simulink model "New_FMS"  (R2018b)
settings: configuration reference "fms_config" (kept outside this file)
values from neighbouring files (symbols this model uses):
  FMS_PARAM = Simulink.Parameter(FMS_PARAM_VALUE)    [fms_model_init.m]
undefined symbols (not defined in the file or in its folder): actuator_cmd, ControlMode, DiscIntNeverNeededParam, FMS_Cmd, mode, MotionState, p_cmd, phi_cmd, PilotMode, psi_rate_cmd, q_cmd, r_cmd, reset, status, theta_cmd, throttle_cmd, u_cmd, v_cmd, VehicleStatus, w_cmd
libraries: FMT_Model_Lib x18, simulink x16
(part 1 of 3)
settings Model: Creator=jiachi  LastModifiedBy=jiachi
settings ConfigSetRef: SourceLocation=Base Workspace

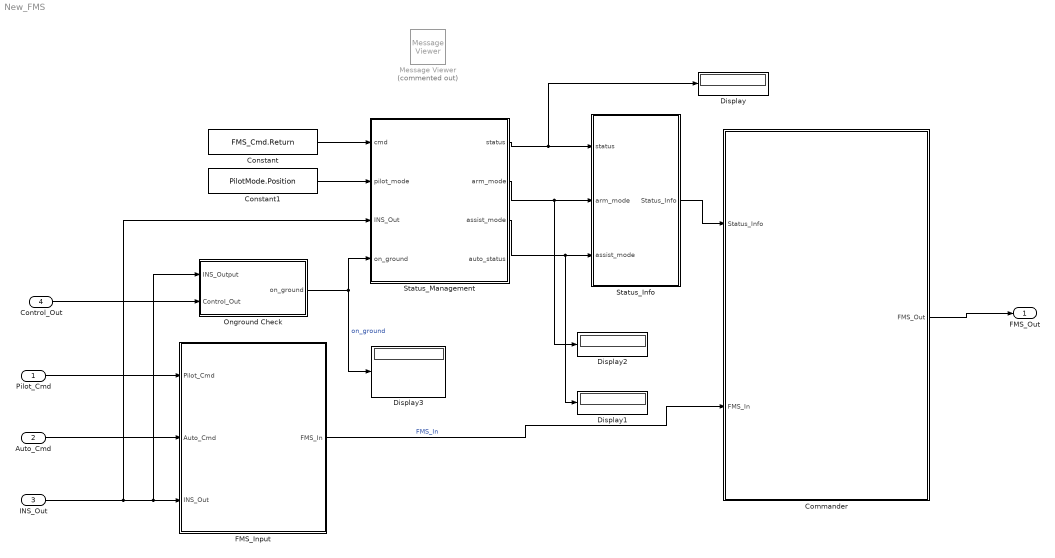
== system New_FMS ==
  Pilot_Cmd : Inport  OutDataTypeStr=Bus: Pilot_Cmd_Bus
  Auto_Cmd : Inport  Port=2  OutDataTypeStr=Bus: Auto_Cmd_Bus
  INS_Out : Inport  Port=3  OutDataTypeStr=Bus: INS_Out_Bus
  Control_Out : Inport  Port=4  OutDataTypeStr=Bus: Control_Out_Bus
  Commander : Subsystem
  Constant : Constant  Value=FMS_Cmd.Return  OutDataTypeStr=Enum: FMS_Cmd
  Constant1 : Constant  Value=PilotMode.Position  OutDataTypeStr=Enum: PilotMode
  Display{,1..3} (4 alike) : Display
  FMS_Input : Subsystem
  Message Viewer : MessageViewer  Commented=on  SavedRootId=#
  Onground Check : Subsystem
  Status_Info : Subsystem
  Status_Management : Stateflow chart  TreatAsAtomicUnit=on
  FMS_Out : Outport  OutDataTypeStr=Bus: FMS_Out_Bus
  wires:
  Status_Management/1(status) -> Status_Info/1(status), Display/1
  Constant/1 -> Status_Management/1(cmd)
  Commander/1(FMS_Out) -> FMS_Out/1
  Constant1/1 -> Status_Management/2(pilot_mode)
  Status_Management/2(arm_mode) -> Display2/1, Status_Info/2(arm_mode)
  Status_Management/3(assist_mode) -> Display1/1, Status_Info/3(assist_mode)
  Pilot_Cmd/1 -> FMS_Input/1(Pilot_Cmd)
  Auto_Cmd/1 -> FMS_Input/2(Auto_Cmd)
  INS_Out/1 -> Status_Management/3(INS_Out), Onground Check/1(INS_Output), FMS_Input/3(INS_Out)
  FMS_Input/1(FMS_In) -> Commander/2(FMS_In)  "FMS_In"
  Status_Info/1(Status_Info) -> Commander/1(Status_Info)
  Control_Out/1 -> Onground Check/2(Control_Out)
  Onground Check/1(on_ground) -> Display3/1, Status_Management/4(on_ground)  "on_ground"

== system New_FMS/Commander ==
  In Bus Element{3..4,6,9} (4 alike) : Inport  PortName=Status_Info
  In Bus Element2 : Inport  PortName=Status_Info  Element=vehicle_status
  In Bus Element{1,5,7..8} (4 alike) : Inport  Port=2  PortName=FMS_In
  Arm : Subsystem  TreatAsAtomicUnit=on
  Disarm : Subsystem  TreatAsAtomicUnit=on
  Land : Subsystem  TreatAsAtomicUnit=on
  Merge : Merge  Inputs=7
  Return : Subsystem  TreatAsAtomicUnit=on
  Standby : Subsystem  TreatAsAtomicUnit=on
  Status_Switch_Case : SwitchCase  CaseConditions={VehicleStatus.Disarm,VehicleStatus.Standby,VehicleStatus.Arm,VehicleStatus.Takeoff,VehicleStatus.Land,VehicleStatus.Return}
  Takeoff : Subsystem  TreatAsAtomicUnit=on
  Unknown : Subsystem  TreatAsAtomicUnit=on
  FMS_Out : Outport
  wires:
  Arm/1(FMS_Out) -> Merge/3
  Status_Switch_Case/6 -> Return/Action
  Takeoff/1(FMS_Out) -> Merge/4
  Status_Switch_Case/7 -> Unknown/Action
  Status_Switch_Case/2 -> Standby/Action
  Land/1(FMS_Out) -> Merge/5
  Unknown/1(FMS_Out) -> Merge/7
  Merge/1 -> FMS_Out/1
  Status_Switch_Case/1 -> Disarm/Action
  Status_Switch_Case/3 -> Arm/Action
  Status_Switch_Case/5 -> Land/Action
  Return/1(FMS_Out) -> Merge/6
  Status_Switch_Case/4 -> Takeoff/Action
  Disarm/1(FMS_Out) -> Merge/1
  Standby/1(FMS_Out) -> Merge/2
  In Bus Element3/1 -> Arm/1(Stauts_Info)
  In Bus Element1/1 -> Arm/2(FMS_In)
  In Bus Element2/1 -> Status_Switch_Case/1
  In Bus Element4/1 -> Takeoff/1(Status_Info)
  In Bus Element5/1 -> Takeoff/2(FMS_In)
  In Bus Element6/1 -> Land/1(Status_Info)
  In Bus Element7/1 -> Land/2(FMS_In)
  In Bus Element8/1 -> Return/2(FMS_In)
  In Bus Element9/1 -> Return/1(Status_Info)

== system New_FMS/FMS_Input ==
  Pilot_Cmd : Inport
  Auto_Cmd : Inport  Port=2
  INS_Out : Inport  Port=3
  Bus Creator : BusCreator  Inputs=4
  Bus Selector : BusSelector  OutputSignals=psi
  Pilot_Cmd_Process : Subsystem
  Psi To DCM : FMT_Model_Lib/Transformation/Psi To DCM
      settings: SourceProductName=FMT Toolbox
  Signal Copy : SignalConversion  OverrideOpt=off
  Signal Copy1 : SignalConversion  OverrideOpt=off
  FMS_In : Outport
  wires:
  Bus Creator/1 -> FMS_In/1
  Pilot_Cmd/1 -> Pilot_Cmd_Process/1(Pilot_Cmd)
  Auto_Cmd/1 -> Signal Copy/1
  INS_Out/1 -> Bus Selector/1, Signal Copy1/1  "INS_Out"
  Pilot_Cmd_Process/1(Pilot_Cmd_Proc) -> Bus Creator/1  "Pilot_Cmd_Proc"
  Bus Selector/1 -> Psi To DCM/1  "<psi>"
  Psi To DCM/1 -> Bus Creator/4  "M_CO"
  Signal Copy/1 -> Bus Creator/2  "Auto_Cmd"
  Signal Copy1/1 -> Bus Creator/3  "INS_Out"

== system New_FMS/Onground Check ==
  INS_Output : Inport
  Control_Out : Inport  Port=2
  Bus Selector1 : BusSelector  OutputSignals=actuator_cmd
  Bus Selector3 : BusSelector  OutputSignals=ax,ay,az
  Compare To Constant : simulink/Logic and Bit Operations/Compare To Constant  relop=<  const=1200  OutDataTypeStr=boolean
  Constant : Constant  Value=4  OutDataTypeStr=uint16
  Divide : Product  Inputs=*/
  First Order LPF : FMT_Model_Lib/Filter/First Order LPF  fc=1/(2*pi*0.5)
      settings: SourceProductName=FMT Toolbox
  First Order LPF1 : FMT_Model_Lib/Filter/First Order LPF  fc=1/(2*pi*0.1)
      settings: SourceProductName=FMT Toolbox
  Interval Test : simulink/Logic and Bit Operations/Interval Test  IntervalClosedRight=on  uplimit=[0.5, 0.5, -9.806+0.5]  IntervalClosedLeft=on  lowlimit=[-0.5, -0.5, -9.806-0.5]  OutDataTypeStr=boolean
  Logical Operator : Logic  Inputs=1  AllPortsSameDT=off  OutDataTypeStr=boolean
  Logical Operator1 : Logic  AllPortsSameDT=off  OutDataTypeStr=boolean
  Matrix Concatenate3 : Concatenate  NumInputs=3  ConcatenateDimension=2
  Selector : Selector  InputPortWidth=16  IndexOptions=Index vector (dialog)  Indices=[1:4]  OutputSizes=1
  Sum of Elements : Sum  Inputs=+
  sample_valid : Subsystem
  on_ground : Outport
  wires:
  Bus Selector3/2 -> Matrix Concatenate3/2  "<ay>"
  Compare To Constant/1 -> Logical Operator1/2
  Bus Selector3/3 -> Matrix Concatenate3/3  "<az>"
  Bus Selector1/1 -> Selector/1  "<actuator_cmd>"
  Bus Selector3/1 -> Matrix Concatenate3/1  "<ax>"
  Selector/1 -> Sum of Elements/1
  INS_Output/1 -> Bus Selector3/1
  Logical Operator1/1 -> sample_valid/1(valid)
  Control_Out/1 -> Bus Selector1/1
  Matrix Concatenate3/1 -> First Order LPF/1
  Interval Test/1 -> Logical Operator/1
  Sum of Elements/1 -> Divide/1
  Constant/1 -> Divide/2
  First Order LPF/1 -> Interval Test/1
  Divide/1 -> First Order LPF1/1
  First Order LPF1/1 -> Compare To Constant/1
  Logical Operator/1 -> Logical Operator1/1
  sample_valid/1(sample_valid) -> on_ground/1

== system New_FMS/Status_Info ==
  status : Inport
  arm_mode : Inport  Port=2
  assist_mode : Inport  Port=3
  Bus Creator : BusCreator  Inputs=3
  Signal Copy : SignalConversion  OverrideOpt=off
  Signal Copy1 : SignalConversion  OverrideOpt=off
  Signal Copy2 : SignalConversion  OverrideOpt=off
  Status_Info : Outport
  wires:
  status/1 -> Signal Copy/1
  arm_mode/1 -> Signal Copy1/1
  assist_mode/1 -> Signal Copy2/1
  Signal Copy/1 -> Bus Creator/1  "vehicle_status"
  Signal Copy1/1 -> Bus Creator/2  "arm_mode"
  Signal Copy2/1 -> Bus Creator/3  "assist_mode"
  Bus Creator/1 -> Status_Info/1

== system New_FMS/Commander/Arm ==
  In Bus Element2 : Inport  PortName=Stauts_Info
  In Bus Element : Inport  PortName=Stauts_Info  Element=arm_mode
  In Bus Element1 : Inport  Port=2  PortName=FMS_In
  Action Port : ActionPort  InitializeStates=reset  ActionType=case
  Assist : Subsystem  TreatAsAtomicUnit=on
  Auto : Subsystem  TreatAsAtomicUnit=on
  Manual : Subsystem  TreatAsAtomicUnit=on
  Merge : Merge  Inputs=4
  Switch Case : SwitchCase  CaseConditions={ArmMode.Manual, ArmMode.Assist, ArmMode.Auto}
  Unknown : Subsystem  TreatAsAtomicUnit=on
  FMS_Out : Outport
  wires:
  Merge/1 -> FMS_Out/1
  In Bus Element/1 -> Switch Case/1
  Switch Case/1 -> Manual/Action
  Switch Case/2 -> Assist/Action
  Switch Case/3 -> Auto/Action
  Switch Case/4 -> Unknown/Action
  Manual/1(FMS_Out) -> Merge/1
  Assist/1(FMS_Out) -> Merge/2
  Auto/1(FMS_Out) -> Merge/3
  Unknown/1(FMS_Out) -> Merge/4
  In Bus Element2/1 -> Assist/1(Stauts_Info)
  In Bus Element1/1 -> Assist/2(FMS_In)

== system New_FMS/Commander/Disarm ==
  Action Port : ActionPort  InitializeStates=reset  ActionType=case
  Bus Assignment : BusAssignment  AssignedSignals=reset,status,actuator_cmd
  Constant : Constant  Value=0  OutDataTypeStr=Bus: FMS_Out_Bus
  Constant1 : Constant  Value=VehicleStatus.Disarm  OutDataTypeStr=Inherit: Inherit via back propagation
  Constant2 : Constant  OutDataTypeStr=Inherit: Inherit via back propagation
  Constant3 : Constant  Value=[1000;1000;1000;1000]  VectorParams1D=off  OutDataTypeStr=Inherit: Inherit via back propagation
  Constant4 : Constant  Value=zeros(12,1)  OutDataTypeStr=Inherit: Inherit via back propagation
  Mux : Mux  Inputs=2
  FMS_Out : Outport
  wires:
  Constant/1 -> Bus Assignment/1
  Bus Assignment/1 -> FMS_Out/1
  Constant2/1 -> Bus Assignment/2
  Constant1/1 -> Bus Assignment/3
  Constant3/1 -> Mux/1
  Constant4/1 -> Mux/2
  Mux/1 -> Bus Assignment/4

== system New_FMS/Commander/Land ==
  In Bus Element4 : Inport  PortName=Status_Info  Element=vehicle_status
  In Bus Element1 : Inport  Port=2  PortName=FMS_In
  Action Port : ActionPort  InitializeStates=reset  ActionType=case
  Bus Assignment1 : BusAssignment  AssignedSignals=reset,status,mode,psi_rate_cmd,u_cmd,v_cmd,w_cmd
  Constant : Constant  Value=0  OutDataTypeStr=Inherit: Inherit via back propagation
  Constant1 : Constant  Value=0  OutDataTypeStr=Bus: FMS_Out_Bus
  Constant2 : Constant  Value=ControlMode.POSCTL  OutDataTypeStr=Inherit: Inherit via back propagation
  Constant3 : Constant  Value=0  OutDataTypeStr=Inherit: Inherit via back propagation
  Constant4 : Constant  Value=0.5  OutDataTypeStr=Inherit: Inherit via back propagation
  Constant5 : Constant  Value=[0; 0]  OutDataTypeStr=single
  Position Command : Subsystem
  FMS_Out : Outport
  wires:
  Constant1/1 -> Bus Assignment1/1
  Constant/1 -> Bus Assignment1/5
  Position Command/2(v_cmd_mPs) -> Bus Assignment1/7
  In Bus Element1/1 -> Position Command/1(FMS_In)
  In Bus Element4/1 -> Bus Assignment1/3
  Constant2/1 -> Bus Assignment1/4
  Constant3/1 -> Bus Assignment1/2
  Position Command/1(u_cmd_mPs) -> Bus Assignment1/6
  Bus Assignment1/1 -> FMS_Out/1
  Constant4/1 -> Bus Assignment1/8
  Constant5/1 -> Position Command/2(home_xy_R)

== system New_FMS/Commander/Return ==
  In Bus Element4 : Inport  PortName=Status_Info  Element=vehicle_status
  In Bus Element : Inport  Port=2  PortName=FMS_In
  In Bus Element3 : Inport  Port=2  PortName=FMS_In
  Action Port : ActionPort  InitializeStates=reset  ActionType=case
  Bus Assignment1 : BusAssignment  AssignedSignals=reset,status,mode,u_cmd,v_cmd,w_cmd,psi_rate_cmd
  Constant2 : Constant  Value=0  OutDataTypeStr=Bus: FMS_Out_Bus
  Constant3 : Constant  Value=ControlMode.POSCTL  OutDataTypeStr=Inherit: Inherit via back propagation
  Constant4 : Constant  Value=0  OutDataTypeStr=Inherit: Inherit via back propagation
  Heading Commander : Subsystem
  L1 : Constant  Value=10  OutDataTypeStr=single
  Subsystem : Subsystem
  Sum : Sum  Inputs=+-|
  Velocity Commander : Subsystem
  FMS_Out : Outport
  wires:
  Bus Assignment1/1 -> FMS_Out/1
  In Bus Element/1 -> Subsystem/1(In1)
  Constant4/1 -> Bus Assignment1/2
  Constant3/1 -> Bus Assignment1/4
  In Bus Element4/1 -> Bus Assignment1/3
  Constant2/1 -> Bus Assignment1/1
  Subsystem/1(P1) -> Sum/2, Velocity Commander/1(P1)
  Subsystem/2(P2) -> Velocity Commander/2(P2), Sum/1
  Subsystem/3(P3) -> Velocity Commander/3(P3)
  L1/1 -> Velocity Commander/4(L1)
  Velocity Commander/1(u_cmd) -> Bus Assignment1/5
  Velocity Commander/2(v_cmd) -> Bus Assignment1/6
  Velocity Commander/3(w_cmd) -> Bus Assignment1/7
  In Bus Element3/1 -> Heading Commander/2(FMS_In), Velocity Commander/5(FMS_In)
  Heading Commander/1(psi_rad_cmd) -> Bus Assignment1/8
  Sum/1 -> Heading Commander/1(P1P2)  "P1P2"

== system New_FMS/Commander/Standby ==
  Action Port : ActionPort  InitializeStates=reset  ActionType=case
  Bus Assignment : BusAssignment  AssignedSignals=reset,status,actuator_cmd
  Constant : Constant  Value=0  OutDataTypeStr=Bus: FMS_Out_Bus
  Constant1 : Constant  Value=VehicleStatus.Standby  OutDataTypeStr=Inherit: Inherit via back propagation
  Constant2 : Constant  OutDataTypeStr=Inherit: Inherit via back propagation
  Constant3 : Constant  Value=[1150;1150;1150;1150]  VectorParams1D=off  OutDataTypeStr=Inherit: Inherit via back propagation
  Constant4 : Constant  Value=zeros(12,1)  OutDataTypeStr=Inherit: Inherit via back propagation
  Mux : Mux  Inputs=2
  FMS_Out : Outport
  wires:
  Constant1/1 -> Bus Assignment/3
  Constant3/1 -> Mux/1
  Mux/1 -> Bus Assignment/4
  Constant4/1 -> Mux/2
  Bus Assignment/1 -> FMS_Out/1
  Constant2/1 -> Bus Assignment/2
  Constant/1 -> Bus Assignment/1

== system New_FMS/Commander/Takeoff ==
  In Bus Element4 : Inport  PortName=Status_Info  Element=vehicle_status
  In Bus Element1 : Inport  Port=2  PortName=FMS_In
  Action Port : ActionPort  InitializeStates=reset  ActionType=case
  Bus Assignment1 : BusAssignment  AssignedSignals=reset,status,mode,psi_rate_cmd,u_cmd,v_cmd,w_cmd
  Constant : Constant  Value=0  OutDataTypeStr=Inherit: Inherit via back propagation
  Constant1 : Constant  Value=0  OutDataTypeStr=Bus: FMS_Out_Bus
  Constant2 : Constant  Value=ControlMode.POSCTL  OutDataTypeStr=Inherit: Inherit via back propagation
  Constant3 : Constant  Value=0  OutDataTypeStr=Inherit: Inherit via back propagation
  Constant4 : Constant  Value=-0.5  OutDataTypeStr=Inherit: Inherit via back propagation
  Position Command : Subsystem
  FMS_Out : Outport
  wires:
  Bus Assignment1/1 -> FMS_Out/1
  Constant1/1 -> Bus Assignment1/1
  Constant/1 -> Bus Assignment1/5
  Constant3/1 -> Bus Assignment1/2
  In Bus Element4/1 -> Bus Assignment1/3
  Constant2/1 -> Bus Assignment1/4
  Position Command/1(u_cmd_mPs) -> Bus Assignment1/6
  Position Command/2(v_cmd_mPs) -> Bus Assignment1/7
  In Bus Element1/1 -> Position Command/1(FMS_In)
  Constant4/1 -> Bus Assignment1/8

== system New_FMS/Commander/Unknown ==
  Action Port : ActionPort  InitializeStates=reset  ActionType=default
  Bus Assignment : BusAssignment  AssignedSignals=reset,status,actuator_cmd
  Constant : Constant  Value=0  OutDataTypeStr=Bus: FMS_Out_Bus
  Constant1 : Constant  Value=VehicleStatus.Disarm  OutDataTypeStr=Inherit: Inherit via back propagation
  Constant2 : Constant  OutDataTypeStr=Inherit: Inherit via back propagation
  Constant3 : Constant  Value=[1000;1000;1000;1000]  VectorParams1D=off  OutDataTypeStr=Inherit: Inherit via back propagation
  Constant4 : Constant  Value=zeros(12,1)  OutDataTypeStr=Inherit: Inherit via back propagation
  Mux : Mux  Inputs=2
  FMS_Out : Outport
  wires:
  Constant/1 -> Bus Assignment/1
  Bus Assignment/1 -> FMS_Out/1
  Constant2/1 -> Bus Assignment/2
  Constant1/1 -> Bus Assignment/3
  Constant3/1 -> Mux/1
  Constant4/1 -> Mux/2
  Mux/1 -> Bus Assignment/4

== system New_FMS/FMS_Input/Pilot_Cmd_Process ==
  Pilot_Cmd : Inport
  Bus Creator : BusCreator  Inputs=8
  Bus Selector : BusSelector  OutputSignals=timestamp,mode,cmd_1,cmd_2,ls_lr,ls_ud,rs_lr,rs_ud
  Saturation{,1..3} (4 alike) : Saturate  UpperLimit=1  LowerLimit=-1
  Signal Copy{,1..3} (4 alike) : SignalConversion  OverrideOpt=off
  Pilot_Cmd_Proc : Outport
  wires:
  Pilot_Cmd/1 -> Bus Selector/1
  Bus Selector/1 -> Signal Copy/1  "<timestamp>"
  Signal Copy/1 -> Bus Creator/1  "timestamp_ms"
  Bus Selector/2 -> Signal Copy1/1  "<mode>"
  Signal Copy1/1 -> Bus Creator/2  "pilot_mode"
  Bus Selector/3 -> Signal Copy2/1  "<cmd_1>"
  Signal Copy2/1 -> Bus Creator/3  "event_cmd"
  Bus Selector/4 -> Signal Copy3/1  "<cmd_2>"
  Signal Copy3/1 -> Bus Creator/4  "stataus_cmd"
  Bus Selector/5 -> Saturation/1  "<ls_lr>"
  Bus Selector/6 -> Saturation1/1  "<ls_ud>"
  Bus Selector/7 -> Saturation2/1  "<rs_lr>"
  Bus Selector/8 -> Saturation3/1  "<rs_ud>"
  Saturation/1 -> Bus Creator/5  "stick_yaw"
  Saturation1/1 -> Bus Creator/6  "stick_throttle"
  Saturation2/1 -> Bus Creator/7  "stick_roll"
  Saturation3/1 -> Bus Creator/8  "stick_pitch"
  Bus Creator/1 -> Pilot_Cmd_Proc/1

== system New_FMS/Onground Check/sample_valid ==
  valid : Inport
  Add : Sum  AccumDataTypeStr=uint32
  Data Type Conversion : DataTypeConversion  OutDataTypeStr=uint32
  Delay : Delay  DelayLength=1  InitialCondition=0  ExternalReset=Falling
      settings: InputPortMap=u0,r5
  Saturation : Saturate  UpperLimit=10000  LowerLimit=0
  valid_samples : simulink/Logic and Bit Operations/Compare To Constant  relop=>  const=100  OutDataTypeStr=boolean
  sample_valid : Outport
  wires:
  Add/1 -> Saturation/1
  valid_samples/1 -> sample_valid/1
  Delay/1 -> Add/2
  valid/1 -> Data Type Conversion/1
  Data Type Conversion/1 -> Delay/2, Add/1
  Saturation/1 -> valid_samples/1, Delay/1

== system New_FMS/Commander/Arm/Assist ==
  In Bus Element{3..5,7,9} (5 alike) : Inport  PortName=Stauts_Info
  In Bus Element : Inport  PortName=Stauts_Info  Element=assist_mode
  In Bus Element{1..2,6,8} (4 alike) : Inport  Port=2  PortName=FMS_In
  Action Port : ActionPort  InitializeStates=reset  ActionType=case
  Acro : Subsystem  TreatAsAtomicUnit=on
  Altitude : Subsystem  TreatAsAtomicUnit=on
  Merge : Merge  Inputs=5
  Position : Subsystem  TreatAsAtomicUnit=on
  Stabilize : Subsystem  TreatAsAtomicUnit=on
  Switch Case : SwitchCase  CaseConditions={AssistMode.Acro, AssistMode.Stabilize, AssistMode.Altitude, AssistMode.Position}
  Unknown : Subsystem  TreatAsAtomicUnit=on
  FMS_Out : Outport
  wires:
  Merge/1 -> FMS_Out/1
  In Bus Element/1 -> Switch Case/1
  Switch Case/1 -> Acro/Action
  Switch Case/2 -> Stabilize/Action
  Switch Case/3 -> Altitude/Action
  Switch Case/4 -> Position/Action
  Switch Case/5 -> Unknown/Action
  Acro/1(FMS_Out) -> Merge/1
  Stabilize/1(FMS_Out) -> Merge/2
  Altitude/1(FMS_Out) -> Merge/3
  Position/1(FMS_Out) -> Merge/4
  Unknown/1(FMS_Out) -> Merge/5
  In Bus Element1/1 -> Stabilize/2(FMS_In)
  In Bus Element2/1 -> Altitude/2(FMS_In)
  In Bus Element3/1 -> Stabilize/1(Status_Info)
  In Bus Element4/1 -> Altitude/1(Status_Info)
  In Bus Element5/1 -> Position/1(Status_Info)
  In Bus Element6/1 -> Position/2(FMS_In)
  In Bus Element7/1 -> Acro/1(Status_Info)
  In Bus Element8/1 -> Acro/2(FMS_In)
  In Bus Element9/1 -> Unknown/1(Status_Info)

== system New_FMS/Commander/Arm/Auto ==
  Action Port : ActionPort  InitializeStates=reset  ActionType=case
  Bus Assignment : BusAssignment  AssignedSignals=reset,status,actuator_cmd
  Constant : Constant  Value=0  OutDataTypeStr=Bus: FMS_Out_Bus
  FMS_Out : Outport
  wires:
  Constant/1 -> Bus Assignment/1
  Bus Assignment/1 -> FMS_Out/1

== system New_FMS/Commander/Arm/Manual ==
  Action Port : ActionPort  InitializeStates=reset  ActionType=case
  Bus Assignment : BusAssignment  AssignedSignals=reset,status,actuator_cmd
  Constant : Constant  Value=0  OutDataTypeStr=Bus: FMS_Out_Bus
  FMS_Out : Outport
  wires:
  Constant/1 -> Bus Assignment/1
  Bus Assignment/1 -> FMS_Out/1

== system New_FMS/Commander/Arm/Unknown ==
  Action Port : ActionPort  InitializeStates=reset  ActionType=default
  Bus Assignment : BusAssignment  AssignedSignals=reset,status,actuator_cmd
  Constant : Constant  Value=0  OutDataTypeStr=Bus: FMS_Out_Bus
  FMS_Out : Outport
  wires:
  Bus Assignment/1 -> FMS_Out/1
  Constant/1 -> Bus Assignment/1

== system New_FMS/Commander/Land/Position Command ==
  FMS_In : Inport
  home_xy_R : Inport  Port=2
  Demux : Demux  Outputs=2
  Position Control : Subsystem
  Saturation1 : Saturate  UpperLimit=FMS_PARAM.VEL_XY_LIM  LowerLimit=-FMS_PARAM.VEL_XY_LIM
  u_cmd_mPs : Outport
  v_cmd_mPs : Outport  Port=2
  wires:
  FMS_In/1 -> Position Control/1(FMS_In)
  Saturation1/1 -> Demux/1
  Demux/1 -> u_cmd_mPs/1
  Demux/2 -> v_cmd_mPs/1
  Position Control/1(uv_cmd_mPs) -> Saturation1/1
  home_xy_R/1 -> Position Control/2(home_xy_R)

== system New_FMS/Commander/Return/Heading Commander ==
  P1P2 : Inport
  FMS_In : Inport  Port=2
  Heading Control : Subsystem
  Included Angle : Subsystem
  North : Constant  Value=[1 0]  OutDataTypeStr=single
  psi_rad_cmd : Outport
  wires:
  Heading Control/1(psi_rate_cmd_radPs) -> psi_rad_cmd/1
  Included Angle/1(angle_rad) -> Heading Control/2(psi_cmd_rad)
  North/1 -> Included Angle/1(vec1)
  FMS_In/1 -> Heading Control/1(FMS_In)
  P1P2/1 -> Included Angle/2(vec2)

== system New_FMS/Commander/Return/Subsystem ==
  In1 : Inport
  Bus Selector : BusSelector  OutputSignals=INS_Out.x_R,INS_Out.y_R
  Constant1 : Constant  Value=[0 0]  OutDataTypeStr=single
  Delay : Delay  DelayLength=1  InitialConditionSource=Input port
      settings: InputPortMap=u0,p4
  Mux : Mux  Inputs=2
  P1 : Outport
  P2 : Outport  Port=2
  P3 : Outport  Port=3
  wires:
  Constant1/1 -> P2/1  "P2"
  In1/1 -> Bus Selector/1
  Delay/1 -> P1/1, Delay/1  "P1"
  Mux/1 -> P3/1, Delay/2  "P3"
  Bus Selector/1 -> Mux/1  "<x_R>"
  Bus Selector/2 -> Mux/2  "<y_R>"

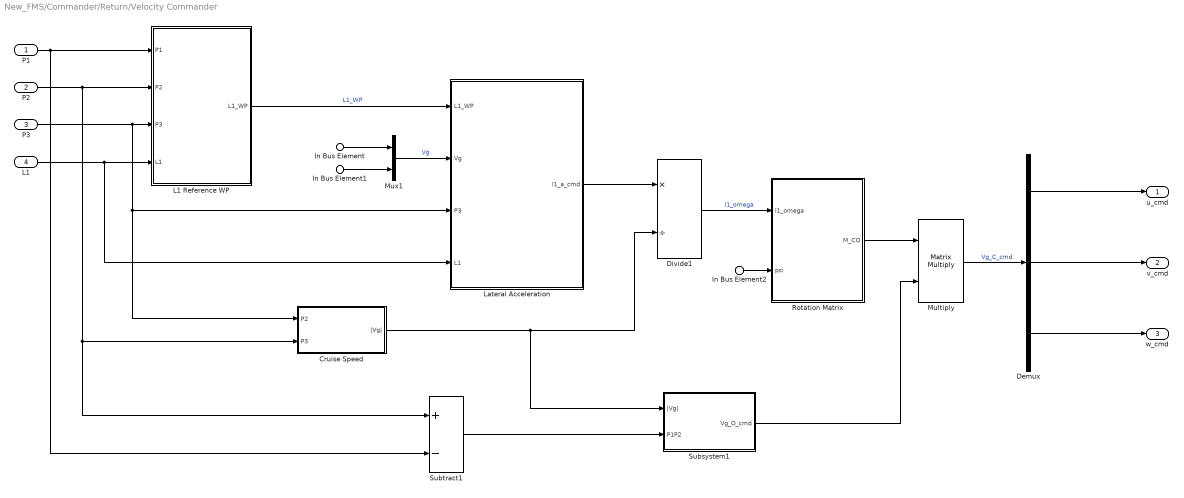
== system New_FMS/Commander/Return/Velocity Commander ==
  P1 : Inport
  P2 : Inport  Port=2
  P3 : Inport  Port=3
  L1 : Inport  Port=4
  In Bus Element : Inport  Port=5  PortName=FMS_In  Element=INS_Out.vn
  In Bus Element1 : Inport  Port=5  PortName=FMS_In  Element=INS_Out.ve
  In Bus Element2 : Inport  Port=5  PortName=FMS_In  Element=INS_Out.psi
  "Cruise Speed " : Subsystem
  Demux : Demux  Outputs=3
  Divide1 : Product  Inputs=*/
  L1 Reference WP : Subsystem
  Lateral Acceleration : Subsystem
  Multiply : Product  Multiplication=Matrix(*)
  Mux1 : Mux  Inputs=2
  Rotation Matrix : Subsystem
  Subsystem1 : Subsystem
  Subtract1 : Sum  Inputs=+-
  u_cmd : Outport
  v_cmd : Outport  Port=2
  w_cmd : Outport  Port=3
  wires:
  "Cruise Speed "/1(|Vg|) -> Divide1/2, Subsystem1/1(|Vg|)
  In Bus Element2/1 -> Rotation Matrix/2(psi)
  L1/1 -> L1 Reference WP/4(L1), Lateral Acceleration/4(L1)
  P1/1 -> Subtract1/2, L1 Reference WP/1(P1)
  L1 Reference WP/1(L1_WP) -> Lateral Acceleration/1(L1_WP)  "L1_WP"
  In Bus Element/1 -> Mux1/1
  Rotation Matrix/1(M_CO) -> Multiply/1
  Multiply/1 -> Demux/1  "Vg_C_cmd"
  Demux/1 -> u_cmd/1
  Demux/3 -> w_cmd/1
  Demux/2 -> v_cmd/1
  P2/1 -> L1 Reference WP/2(P2), Subtract1/1, "Cruise Speed "/2(P3)
  Mux1/1 -> Lateral Acceleration/2(Vg)  "Vg"
  Divide1/1 -> Rotation Matrix/1(l1_omega)  "l1_omega"
  In Bus Element1/1 -> Mux1/2
  P3/1 -> Lateral Acceleration/3(P3), "Cruise Speed "/1(P2), L1 Reference WP/3(P3)
  Subsystem1/1(Vg_O_cmd) -> Multiply/2
  Subtract1/1 -> Subsystem1/2(P1P2)
  Lateral Acceleration/1(l1_a_cmd) -> Divide1/1

== system New_FMS/Commander/Takeoff/Position Command ==
  FMS_In : Inport
  Constant : Constant  Value=MotionState.Hold  OutDataTypeStr=Enum: MotionState
  Controller : Subsystem
  Demux : Demux  Outputs=2
  u_cmd_mPs : Outport
  v_cmd_mPs : Outport  Port=2
  wires:
  FMS_In/1 -> Controller/2(FMS_In)
  Controller/1(uv_cmd_mPs) -> Demux/1
  Demux/1 -> u_cmd_mPs/1
  Demux/2 -> v_cmd_mPs/1
  Constant/1 -> Controller/1(motion_state)

== system New_FMS/Commander/Arm/Assist/Acro ==
  In Bus Element4 : Inport  PortName=Status_Info  Element=vehicle_status
  In Bus Element2 : Inport  Port=2  PortName=FMS_In  Element=Pilot_Cmd_Proc.stick_throttle
  In Bus Element1 : Inport  Port=2  PortName=FMS_In  Element=Pilot_Cmd_Proc.stick_pitch
  In Bus Element3 : Inport  Port=2  PortName=FMS_In  Element=Pilot_Cmd_Proc.stick_roll
  In Bus Element5 : Inport  Port=2  PortName=FMS_In  Element=Pilot_Cmd_Proc.stick_yaw
  Action Port : ActionPort  InitializeStates=reset  ActionType=case
  Angular Rate Command : Subsystem
  Bus Assignment : BusAssignment  AssignedSignals=reset,status,mode,p_cmd,q_cmd,r_cmd,throttle_cmd
  Constant : Constant  Value=0  OutDataTypeStr=Bus: FMS_Out_Bus
  Constant1 : Constant  Value=0  OutDataTypeStr=Inherit: Inherit via back propagation
  Constant2 : Constant  Value=ControlMode.Acro  OutDataTypeStr=Inherit: Inherit via back propagation
  Throttle Command : Subsystem
  FMS_Out : Outport
  wires:
  Constant1/1 -> Bus Assignment/2
  Constant2/1 -> Bus Assignment/4
  Angular Rate Command/3(r_cmd_radPs) -> Bus Assignment/7
  Bus Assignment/1 -> FMS_Out/1
  Constant/1 -> Bus Assignment/1
  Angular Rate Command/1(p_cmd_radPs) -> Bus Assignment/5
  Angular Rate Command/2(q_cmd_radPs) -> Bus Assignment/6
  Throttle Command/1(throttle_cmd) -> Bus Assignment/8
  In Bus Element4/1 -> Bus Assignment/3
  In Bus Element2/1 -> Throttle Command/1(stick_throttle)
  In Bus Element5/1 -> Angular Rate Command/3(stick_yaw)
  In Bus Element1/1 -> Angular Rate Command/2(stick_pitch)
  In Bus Element3/1 -> Angular Rate Command/1(stick_roll)

== system New_FMS/Commander/Arm/Assist/Altitude ==
  In Bus Element4 : Inport  PortName=Status_Info  Element=vehicle_status
  In Bus Element3 : Inport  Port=2  PortName=FMS_In
  In Bus Element5 : Inport  Port=2  PortName=FMS_In
  In Bus Element1 : Inport  Port=2  PortName=FMS_In  Element=Pilot_Cmd_Proc.stick_roll
  In Bus Element2 : Inport  Port=2  PortName=FMS_In  Element=Pilot_Cmd_Proc.stick_pitch
  Action Port : ActionPort  InitializeStates=reset  ActionType=case
  Altitude Command : Subsystem
  Attitude Command : Subsystem
  Bus Assignment : BusAssignment  AssignedSignals=reset,status,mode,phi_cmd,theta_cmd,psi_rate_cmd,w_cmd
  Constant : Constant  Value=0  OutDataTypeStr=Bus: FMS_Out_Bus
  Constant2 : Constant  Value=ControlMode.ALTCTL  OutDataTypeStr=Inherit: Inherit via back propagation
  Constant3 : Constant  Value=0  OutDataTypeStr=Inherit: Inherit via back propagation
  Heading Command : Subsystem
  FMS_Out : Outport
  wires:
  Constant/1 -> Bus Assignment/1
  Bus Assignment/1 -> FMS_Out/1
  In Bus Element4/1 -> Bus Assignment/3
  Constant2/1 -> Bus Assignment/4
  In Bus Element1/1 -> Attitude Command/1(stick_roll)
  In Bus Element2/1 -> Attitude Command/2(stick_pitch)
  In Bus Element3/1 -> Heading Command/1(FMS_In)
  Altitude Command/1(w_cmd_mPs) -> Bus Assignment/8
  Constant3/1 -> Bus Assignment/2
  Attitude Command/1(phi_cmd_radPs) -> Bus Assignment/5
  Attitude Command/2(theta_cmd_radPs) -> Bus Assignment/6
  Heading Command/1(psi_rate_cmd_radPs) -> Bus Assignment/7
  In Bus Element5/1 -> Altitude Command/1(FMS_In)

== system New_FMS/Commander/Arm/Assist/Position ==
  In Bus Element4 : Inport  PortName=Status_Info  Element=vehicle_status
  In Bus Element3 : Inport  Port=2  PortName=FMS_In
  In Bus Element5 : Inport  Port=2  PortName=FMS_In
  In Bus Element1 : Inport  Port=2  PortName=FMS_In
  Action Port : ActionPort  InitializeStates=reset  ActionType=case
  Altitude Command : Subsystem
  Bus Assignment : BusAssignment  AssignedSignals=reset,status,mode,psi_rate_cmd,u_cmd,v_cmd,w_cmd
  Constant : Constant  Value=0  OutDataTypeStr=Bus: FMS_Out_Bus
  Constant2 : Constant  Value=ControlMode.POSCTL  OutDataTypeStr=Inherit: Inherit via back propagation
  Constant3 : Constant  Value=0  OutDataTypeStr=Inherit: Inherit via back propagation
  Heading Command : Subsystem
  Position Command : Subsystem
  FMS_Out : Outport
  wires:
  Bus Assignment/1 -> FMS_Out/1
  Constant/1 -> Bus Assignment/1
  Constant3/1 -> Bus Assignment/2
  In Bus Element4/1 -> Bus Assignment/3
  Constant2/1 -> Bus Assignment/4
  Heading Command/1(psi_rate_cmd_radPs) -> Bus Assignment/5
  In Bus Element3/1 -> Heading Command/1(FMS_In)
  Altitude Command/1(w_cmd_mPs) -> Bus Assignment/8
  In Bus Element5/1 -> Altitude Command/1(FMS_In)
  In Bus Element1/1 -> Position Command/1(FMS_In)
  Position Command/1(u_cmd_mPs) -> Bus Assignment/6
  Position Command/2(v_cmd_mPs) -> Bus Assignment/7

== system New_FMS/Commander/Arm/Assist/Stabilize ==
  In Bus Element4 : Inport  PortName=Status_Info  Element=vehicle_status
  In Bus Element3 : Inport  Port=2  PortName=FMS_In
  In Bus Element1 : Inport  Port=2  PortName=FMS_In  Element=Pilot_Cmd_Proc.stick_roll
  In Bus Element2 : Inport  Port=2  PortName=FMS_In  Element=Pilot_Cmd_Proc.stick_pitch
  In Bus Element : Inport  Port=2  PortName=FMS_In  Element=Pilot_Cmd_Proc.stick_throttle
  Action Port : ActionPort  InitializeStates=reset  ActionType=case
  Attitude Command : Subsystem
  Bus Assignment : BusAssignment  AssignedSignals=reset,status,mode,phi_cmd,theta_cmd,psi_rate_cmd,throttle_cmd
  Constant : Constant  Value=0  OutDataTypeStr=Bus: FMS_Out_Bus
  Constant1 : Constant  Value=0  OutDataTypeStr=Inherit: Inherit via back propagation
  Constant2 : Constant  Value=ControlMode.Stabilize  OutDataTypeStr=Inherit: Inherit via back propagation
  Heading Command : Subsystem
  Throttle Command : Subsystem
  FMS_Out : Outport
  wires:
  Bus Assignment/1 -> FMS_Out/1
  Constant/1 -> Bus Assignment/1
  Constant1/1 -> Bus Assignment/2
  Constant2/1 -> Bus Assignment/4
  Heading Command/1(psi_rate_cmd_radPs) -> Bus Assignment/7
  Attitude Command/1(phi_cmd_radPs) -> Bus Assignment/5
  Attitude Command/2(theta_cmd_radPs) -> Bus Assignment/6
  In Bus Element1/1 -> Attitude Command/1(stick_roll)
  In Bus Element2/1 -> Attitude Command/2(stick_pitch)
  In Bus Element/1 -> Throttle Command/1(stick_throttle)
  Throttle Command/1(throttle_cmd) -> Bus Assignment/8
  In Bus Element3/1 -> Heading Command/1(FMS_In)
  In Bus Element4/1 -> Bus Assignment/3

== system New_FMS/Commander/Arm/Assist/Unknown ==
  In Bus Element4 : Inport  PortName=Status_Info  Element=vehicle_status
  Action Port : ActionPort  InitializeStates=reset  ActionType=default
  Bus Assignment : BusAssignment  AssignedSignals=reset,status,mode,actuator_cmd
  Constant : Constant  Value=0  OutDataTypeStr=Bus: FMS_Out_Bus
  Constant1 : Constant  OutDataTypeStr=Inherit: Inherit via back propagation
  Constant2 : Constant  Value=ControlMode.Unknown  OutDataTypeStr=Inherit: Inherit via back propagation
  Constant3 : Constant  Value=zeros(16,1)  OutDataTypeStr=Inherit: Inherit via back propagation
  FMS_Out : Outport
  wires:
  Constant/1 -> Bus Assignment/1
  Bus Assignment/1 -> FMS_Out/1
  Constant1/1 -> Bus Assignment/2
  Constant2/1 -> Bus Assignment/4
  In Bus Element4/1 -> Bus Assignment/3
  Constant3/1 -> Bus Assignment/5

== system New_FMS/Commander/Land/Position Command/Position Control ==
  FMS_In : Inport
  home_xy_R : Inport  Port=2
  Bus Selector : BusSelector  OutputSignals=INS_Out.psi
  Bus_Selection : Subsystem
  Constant : Constant  Value=0  OutDataTypeStr=Inherit: Inherit via back propagation
  Gain2 : Gain  Gain=FMS_PARAM.XY_P  OutDataTypeStr=single
  Multiply : Product  Multiplication=Matrix(*)
  Mux : Mux  Inputs=2
  Psi To DCM : FMT_Model_Lib/Transformation/Psi To DCM
      settings: SourceProductName=FMT Toolbox
  Selector : Selector  InputPortWidth=3  IndexOptions=Index vector (dialog)  Indices=[1 2]  OutputSizes=1
  Sum : Sum  Inputs=-+|
  uv_cmd_mPs : Outport
  wires:
  Gain2/1 -> uv_cmd_mPs/1
  Bus_Selection/1(xy_R_O_m) -> Sum/1  "xy_est_R"
  Sum/1 -> Mux/1  "xy_err_R"
  home_xy_R/1 -> Sum/2
  FMS_In/1 -> Bus Selector/1, Bus_Selection/1(FMS_In)
  Constant/1 -> Mux/2
  Psi To DCM/1 -> Multiply/1  "M_CO"
  Multiply/1 -> Selector/1
  Mux/1 -> Multiply/2
  Selector/1 -> Gain2/1
  Bus Selector/1 -> Psi To DCM/1  "<psi>"

== system New_FMS/Commander/Return/Heading Commander/Heading Control ==
  FMS_In : Inport
  psi_cmd_rad : Inport  Port=2
  Bus Selector : BusSelector  OutputSignals=INS_Out.psi
  Heading Control : Subsystem  TreatAsAtomicUnit=on
  TD : Subsystem
  psi_rate_cmd_radPs : Outport
  wires:
  TD/1(v1) -> Heading Control/2(psi_cmd_rad)
  FMS_In/1 -> Bus Selector/1, Heading Control/1(FMS_In)
  Bus Selector/1 -> TD/2(v0)  "<psi>"
  Heading Control/1(psi_rate_cmd_radPs) -> psi_rate_cmd_radPs/1
  psi_cmd_rad/1 -> TD/1(v)

== system New_FMS/Commander/Return/Heading Commander/Included Angle ==
  vec1 : Inport
  vec2 : Inport  Port=2
  2D Cross Product : FMT_Model_Lib/Math/2D Cross Product
      settings: SourceProductName=FMT Toolbox
  Acos : Trigonometry  Operator=acos
  Constant4 : Constant  OutDataTypeStr=single
  Demux : Demux  Outputs=2
  Demux1 : Demux  Outputs=2
  Dot Product : DotProduct  InputSameDT=on  OutDataTypeStr=Inherit: Inherit via internal rule
  Multiply : Product
  Mux : Mux  Inputs=2
  Mux1 : Mux  Inputs=2
  Sign1 : Signum
  Switch2 : Switch  Criteria=u2 ~= 0
  Vector Normalize : FMT_Model_Lib/Math/Vector Normalize
      settings: SourceProductName=FMT Toolbox
  Vector Normalize1 : FMT_Model_Lib/Math/Vector Normalize
      settings: SourceProductName=FMT Toolbox
  angle_rad : Outport
  wires:
  Dot Product/1 -> Acos/1
  Demux1/1 -> Mux1/2
  Mux1/1 -> Vector Normalize/1
  Demux1/2 -> Mux1/1
  Sign1/1 -> Switch2/1, Switch2/2
  Vector Normalize1/1 -> Dot Product/2, 2D Cross Product/1
  Demux/2 -> Mux/1
  Vector Normalize/1 -> Dot Product/1, 2D Cross Product/2
  2D Cross Product/1 -> Sign1/1
  Multiply/1 -> angle_rad/1
  vec1/1 -> Demux1/1
  Demux/1 -> Mux/2
  Constant4/1 -> Switch2/3
  vec2/1 -> Demux/1
  Mux/1 -> Vector Normalize1/1
  Acos/1 -> Multiply/1
  Switch2/1 -> Multiply/2

== system New_FMS/Commander/Return/Velocity Commander/Cruise Speed  ==
  P2 : Inport
  P3 : Inport  Port=2
  Gain : Gain  Gain=0.5  OutDataTypeStr=Inherit: Same as input
  Sum : Sum  Inputs=|+-
  Switch : Switch  Criteria=u2 > Threshold  Threshold=10
  Vector Modulus : FMT_Model_Lib/Math/Vector Modulus
      settings: SourceProductName=FMT Toolbox
  vel : Constant  Value=5  OutDataTypeStr=single
  |Vg| : Outport
  wires:
  P2/1 -> Sum/1
  P3/1 -> Sum/2
  Sum/1 -> Vector Modulus/1
  Vector Modulus/1 -> Gain/1, Switch/2
  vel/1 -> Switch/1  "|Vg|"
  Switch/1 -> |Vg|/1
  Gain/1 -> Switch/3

== system New_FMS/Commander/Return/Velocity Commander/L1 Reference WP ==
  P1 : Inport
  P2 : Inport  Port=2
  P3 : Inport  Port=3
  L1 : Inport  Port=4
  Compare To Constant : simulink/Logic and Bit Operations/Compare To Constant  relop=>=  const=0  OutDataTypeStr=boolean
  Compare To Constant1 : simulink/Logic and Bit Operations/Compare To Constant  relop=>  const=0  OutDataTypeStr=boolean
  NearbyRefWP : MATLAB Function  TreatAsAtomicUnit=on
  OutRegionRegWP : MATLAB Function  TreatAsAtomicUnit=on
  SearchL1RefWP : MATLAB Function  TreatAsAtomicUnit=on
  Switch : Switch  Criteria=u2 > Threshold
  Switch1 : Switch  Criteria=u2 > Threshold
  L1_WP : Outport
  wires:
  NearbyRefWP/1(P) -> Switch1/1  "NearbyWP"
  SearchL1RefWP/1(P) -> Switch/1  "L1_Ref_P"
  Switch1/1 -> L1_WP/1
  OutRegionRegWP/1(P) -> Switch/3  "out_WP"
  L1/1 -> NearbyRefWP/3(L1), SearchL1RefWP/4(L1)
  Switch/1 -> Switch1/3
  P3/1 -> OutRegionRegWP/3(P3), SearchL1RefWP/3(P3), NearbyRefWP/2(P3)
  P2/1 -> OutRegionRegWP/2(P2), NearbyRefWP/1(P2), SearchL1RefWP/2(P2)
  P1/1 -> OutRegionRegWP/1(P1), SearchL1RefWP/1(P1)
  Compare To Constant1/1 -> Switch1/2
  SearchL1RefWP/2(u) -> Compare To Constant/1  "l1_u"
  NearbyRefWP/2(d) -> Compare To Constant1/1  "distance"
  Compare To Constant/1 -> Switch/2

== system New_FMS/Commander/Return/Velocity Commander/Lateral Acceleration ==
  L1_WP : Inport
  Vg : Inport  Port=2
  P3 : Inport  Port=3
  L1 : Inport  Port=4
  Divide : Product  Inputs=*/
  Gain : Gain  Gain=2
  Included Angle : Subsystem
  Multiply1 : Product
  Saturation : Saturate  UpperLimit=pi/2  LowerLimit=-pi/2
  Sin : Trigonometry
  Square : Math  Operator=square  SaturateOnIntegerOverflow=on
  Subtract : Sum  Inputs=+-
  Vector Modulus : FMT_Model_Lib/Math/Vector Modulus
      settings: SourceProductName=FMT Toolbox
  Vector Normalize : FMT_Model_Lib/Math/Vector Normalize
      settings: SourceProductName=FMT Toolbox
  Vector Normalize1 : FMT_Model_Lib/Math/Vector Normalize
      settings: SourceProductName=FMT Toolbox
  l1_a_cmd : Outport
  wires:
  P3/1 -> Subtract/2
  Sin/1 -> Multiply1/1  "sin_alpha"
  Vg/1 -> Vector Modulus/1, Vector Normalize/1
  L1/1 -> Divide/2
  Square/1 -> Gain/1
  Vector Normalize1/1 -> Included Angle/2(vec2)
  Divide/1 -> l1_a_cmd/1  "l1_a_cmd"
  Multiply1/1 -> Divide/1
  Vector Normalize/1 -> Included Angle/1(vec1)
  L1_WP/1 -> Subtract/1
  Gain/1 -> Multiply1/2
  Subtract/1 -> Vector Normalize1/1
  Vector Modulus/1 -> Square/1
  Included Angle/1(angle_rad) -> Saturation/1  "L1_alpha"
  Saturation/1 -> Sin/1

== system New_FMS/Commander/Return/Velocity Commander/Rotation Matrix ==
  l1_omega : Inport
  psi : Inport  Port=2
  Add : Sum  Inputs=-+
  Discrete-Time Integrator : DiscreteIntegrator  SampleTime=-1  ICPrevOutput=DiscIntNeverNeededParam  ICPrevScaledInput=DiscIntNeverNeededParam
  Psi To DCM : FMT_Model_Lib/Transformation/Psi To DCM
      settings: SourceProductName=FMT Toolbox
  M_CO : Outport
  wires:
  Psi To DCM/1 -> M_CO/1
  Discrete-Time Integrator/1 -> Add/1
  psi/1 -> Add/2
  l1_omega/1 -> Discrete-Time Integrator/1
  Add/1 -> Psi To DCM/1

== system New_FMS/Commander/Return/Velocity Commander/Subsystem1 ==
  |Vg| : Inport
  P1P2 : Inport  Port=2
  Constant : Constant  Value=0  OutDataTypeStr=single
  Multiply2 : Product
  Mux : Mux  Inputs=2
  Vector Normalize2 : FMT_Model_Lib/Math/Vector Normalize
      settings: SourceProductName=FMT Toolbox
  Vg_O_cmd : Outport
  wires:
  Vector Normalize2/1 -> Multiply2/1
  Multiply2/1 -> Vg_O_cmd/1
  P1P2/1 -> Mux/1
  Mux/1 -> Vector Normalize2/1
  Constant/1 -> Mux/2
  |Vg|/1 -> Multiply2/2

== system New_FMS/Commander/Takeoff/Position Command/Controller ==
  motion_state : Inport
  In Bus Element : Inport  Port=2  PortName=FMS_In
  In Bus Element1 : Inport  Port=2  PortName=FMS_In
  Brake Control : Subsystem  TreatAsAtomicUnit=on
  Hold Control : Subsystem  TreatAsAtomicUnit=on
  Merge : Merge  Inputs=3
  Move Control : Subsystem  TreatAsAtomicUnit=on
  Saturation1 : Saturate  UpperLimit=FMS_PARAM.VEL_XY_LIM  LowerLimit=-FMS_PARAM.VEL_XY_LIM
  Switch Case : SwitchCase  CaseConditions={MotionState.Hold, MotionState.Brake, MotionState.Move}  ShowDefaultCase=off
  uv_cmd_mPs : Outport
  wires:
  Merge/1 -> Saturation1/1
  Saturation1/1 -> uv_cmd_mPs/1
  motion_state/1 -> Switch Case/1
  Switch Case/1 -> Hold Control/Action
  Switch Case/2 -> Brake Control/Action
  Switch Case/3 -> Move Control/Action
  In Bus Element/1 -> Hold Control/1(FMS_In)
  In Bus Element1/1 -> Move Control/1(FMS_In)
  Hold Control/1(uv_cmd_mPs) -> Merge/1
  Brake Control/1(uv_cmd_mPs) -> Merge/2
  Move Control/1(uv_cmd_mPs) -> Merge/3

== system New_FMS/Commander/Arm/Assist/Acro/Angular Rate Command ==
  stick_roll : Inport
  stick_pitch : Inport  Port=2
  stick_yaw : Inport  Port=3
  Gain : Gain  Gain=pi
  Gain1 : Gain  Gain=-pi
  Gain2 : Gain  Gain=pi/2
  p_cmd_radPs : Outport
  q_cmd_radPs : Outport  Port=2
  r_cmd_radPs : Outport  Port=3
  wires:
  stick_roll/1 -> Gain/1
  Gain/1 -> p_cmd_radPs/1
  stick_pitch/1 -> Gain1/1
  stick_yaw/1 -> Gain2/1
  Gain1/1 -> q_cmd_radPs/1
  Gain2/1 -> r_cmd_radPs/1

== system New_FMS/Commander/Arm/Assist/Acro/Throttle Command ==
  stick_throttle : Inport
  Add : Sum
  Constant4 : Constant  OutDataTypeStr=single
  Constant5 : Constant  Value=1000  OutDataTypeStr=uint32
  Gain2 : Gain  Gain=500  OutDataTypeStr=uint32
  Saturation : Saturate  UpperLimit=2  LowerLimit=0
  Sum : Sum  Inputs=|++
  throttle_cmd : Outport
  wires:
  Constant4/1 -> Sum/2
  Add/1 -> throttle_cmd/1
  Constant5/1 -> Add/2
  stick_throttle/1 -> Sum/1
  Saturation/1 -> Gain2/1
  Sum/1 -> Saturation/1
  Gain2/1 -> Add/1

== system New_FMS/Commander/Arm/Assist/Altitude/Altitude Command ==
  FMS_In : Inport
  Controller : Subsystem
  Movement Check : Subsystem
  w_cmd_mPs : Outport
  wires:
  FMS_In/1 -> Movement Check/1(FMS_In), Controller/2(FMS_In)
  Movement Check/1(motion_state) -> Controller/1(motion_state)
  Controller/1(w_cmd_mPs) -> w_cmd_mPs/1

== system New_FMS/Commander/Arm/Assist/Altitude/Attitude Command ==
  stick_roll : Inport
  stick_pitch : Inport  Port=2
  DeadZone : Subsystem  mask{th=FMS_PARAM.ROLL_DZ}
      mask prompts: th "Threshold"
      mask Display: disp('Dead Zone')
  DeadZone2 : Subsystem  mask{th=FMS_PARAM.PITCH_DZ}
      mask prompts: th "Threshold"
      mask Display: disp('Dead Zone')
  Gain : Gain  Gain=FMS_PARAM.ROLL_PITCH_LIM
  Gain1 : Gain  Gain=-FMS_PARAM.ROLL_PITCH_LIM
  Phi_CMD_TD : Subsystem
  Theta_CMD_TD : Subsystem
  phi_cmd_radPs : Outport
  theta_cmd_radPs : Outport  Port=2
  wires:
  DeadZone/1(y) -> Gain/1
  DeadZone2/1(y) -> Gain1/1
  Gain/1 -> Phi_CMD_TD/1(v)
  Gain1/1 -> Theta_CMD_TD/1(v)
  stick_roll/1 -> DeadZone/1(u)
  Phi_CMD_TD/1(v1) -> phi_cmd_radPs/1
  stick_pitch/1 -> DeadZone2/1(u)
  Theta_CMD_TD/1(v1) -> theta_cmd_radPs/1

== system New_FMS/Commander/Arm/Assist/Altitude/Heading Command ==
  FMS_In : Inport
  Controller : Subsystem
  Movement Check : Subsystem
  psi_rate_cmd_radPs : Outport
  wires:
  FMS_In/1 -> Movement Check/1(FMS_In), Controller/2(FMS_In)
  Movement Check/1(motion_state) -> Controller/1(motion_state)
  Controller/1(psi_rate_cmd_radPs) -> psi_rate_cmd_radPs/1

== system New_FMS/Commander/Arm/Assist/Position/Altitude Command ==
  FMS_In : Inport
  Controller : Subsystem
  Movement Check : Subsystem
  w_cmd_mPs : Outport
  wires:
  FMS_In/1 -> Movement Check/1(FMS_In), Controller/2(FMS_In)
  Movement Check/1(motion_state) -> Controller/1(motion_state)
  Controller/1(w_cmd_mPs) -> w_cmd_mPs/1

== system New_FMS/Commander/Arm/Assist/Position/Heading Command ==
  FMS_In : Inport
  Controller : Subsystem
  Movement Check : Subsystem
  psi_rate_cmd_radPs : Outport
  wires:
  FMS_In/1 -> Movement Check/1(FMS_In), Controller/2(FMS_In)
  Movement Check/1(motion_state) -> Controller/1(motion_state)  "head_ms"
  Controller/1(psi_rate_cmd_radPs) -> psi_rate_cmd_radPs/1

== system New_FMS/Commander/Arm/Assist/Position/Position Command ==
  FMS_In : Inport
  Controller : Subsystem
  Demux : Demux  Outputs=2
  Movement Check : Subsystem
  u_cmd_mPs : Outport
  v_cmd_mPs : Outport  Port=2
  wires:
  FMS_In/1 -> Movement Check/1(FMS_In), Controller/2(FMS_In)
  Movement Check/1(motion_state) -> Controller/1(motion_state)
  Controller/1(uv_cmd_mPs) -> Demux/1
  Demux/1 -> u_cmd_mPs/1
  Demux/2 -> v_cmd_mPs/1

== system New_FMS/Commander/Arm/Assist/Stabilize/Attitude Command ==
  stick_roll : Inport
  stick_pitch : Inport  Port=2
  DeadZone : Subsystem  mask{th=FMS_PARAM.ROLL_DZ}
      mask prompts: th "Threshold"
      mask Display: disp('Dead Zone')
  DeadZone2 : Subsystem  mask{th=FMS_PARAM.PITCH_DZ}
      mask prompts: th "Threshold"
      mask Display: disp('Dead Zone')
  Gain : Gain  Gain=FMS_PARAM.ROLL_PITCH_LIM
  Gain1 : Gain  Gain=-FMS_PARAM.ROLL_PITCH_LIM
  Phi_CMD_TD : Subsystem
  Theta_CMD_TD : Subsystem
  phi_cmd_radPs : Outport
  theta_cmd_radPs : Outport  Port=2
  wires:
  DeadZone/1(y) -> Gain/1
  DeadZone2/1(y) -> Gain1/1
  Gain/1 -> Phi_CMD_TD/1(v)
  Gain1/1 -> Theta_CMD_TD/1(v)
  stick_roll/1 -> DeadZone/1(u)
  Phi_CMD_TD/1(v1) -> phi_cmd_radPs/1
  stick_pitch/1 -> DeadZone2/1(u)
  Theta_CMD_TD/1(v1) -> theta_cmd_radPs/1

== system New_FMS/Commander/Arm/Assist/Stabilize/Heading Command ==
  FMS_In : Inport
  Controller : Subsystem
  Movement Check : Subsystem
  psi_rate_cmd_radPs : Outport
  wires:
  FMS_In/1 -> Movement Check/1(FMS_In), Controller/2(FMS_In)
  Movement Check/1(motion_state) -> Controller/1(motion_state)
  Controller/1(psi_rate_cmd_radPs) -> psi_rate_cmd_radPs/1

== system New_FMS/Commander/Arm/Assist/Stabilize/Throttle Command ==
  stick_throttle : Inport
  Add : Sum
  Constant4 : Constant  OutDataTypeStr=single
  Constant5 : Constant  Value=1000  OutDataTypeStr=uint32
  Gain2 : Gain  Gain=500  OutDataTypeStr=uint32
  Saturation : Saturate  UpperLimit=2  LowerLimit=0
  Sum : Sum  Inputs=|++
  throttle_cmd : Outport
  wires:
  Constant4/1 -> Sum/2
  Add/1 -> throttle_cmd/1
  Constant5/1 -> Add/2
  stick_throttle/1 -> Sum/1
  Saturation/1 -> Gain2/1
  Sum/1 -> Saturation/1
  Gain2/1 -> Add/1

== system New_FMS/Commander/Land/Position Command/Position Control/Bus_Selection ==
  FMS_In : Inport
  Bus Selector2 : BusSelector  OutputSignals=INS_Out.x_R,INS_Out.y_R
  Mux : Mux  Inputs=2
  xy_R_O_m : Outport
  wires:
  FMS_In/1 -> Bus Selector2/1
  Bus Selector2/1 -> Mux/1  "<x_R>"
  Mux/1 -> xy_R_O_m/1
  Bus Selector2/2 -> Mux/2  "<y_R>"

== system New_FMS/Commander/Return/Heading Commander/Heading Control/Heading Control ==
  FMS_In : Inport
  psi_cmd_rad : Inport  Port=2
  Bus_Selection : Subsystem
  Gain2 : Gain  Gain=FMS_PARAM.YAW_P  OutDataTypeStr=single
  Saturation : Saturate  UpperLimit=FMS_PARAM.YAW_RATE_LIM  LowerLimit=-FMS_PARAM.YAW_RATE_LIM
  Sum : Sum  Inputs=-+|
  psi_err_saturation : Subsystem
  psi_rate_cmd_radPs : Outport
  wires:
  Gain2/1 -> Saturation/1
  Bus_Selection/1(psi_rad) -> Sum/1  "psi_est_rad"
  psi_err_saturation/1(psi_err_rad) -> Gain2/1
  Sum/1 -> psi_err_saturation/1(psi_err_in)  "psi_error_rad"
  FMS_In/1 -> Bus_Selection/1(FMS_In)
  psi_cmd_rad/1 -> Sum/2
  Saturation/1 -> psi_rate_cmd_radPs/1

== system New_FMS/Commander/Return/Heading Commander/Heading Control/TD ==
  v : Inport
  v0 : Inport  Port=2
  Integrator : DiscreteIntegrator  SampleTime=-1  LimitOutput=on  UpperSaturationLimit=FMS_PARAM.YAW_RATE_LIM  LowerSaturationLimit=-FMS_PARAM.YAW_RATE_LIM  ICPrevOutput=DiscIntNeverNeededParam  ICPrevScaledInput=DiscIntNeverNeededParam
  Integrator1 : DiscreteIntegrator  InitialConditionSource=external  SampleTime=-1  ICPrevOutput=DiscIntNeverNeededParam  ICPrevScaledInput=DiscIntNeverNeededParam
  Subtract : Sum  Inputs=+-
  "fhan " : Subsystem  mask{r0=pi/4, h0=1}
      mask DialogControl ParameterGroupVar Prompt: fhan(v1,v2,r0,h0)
  v1 : Outport
  wires:
  Integrator1/1 -> v1/1, Subtract/1
  v/1 -> Subtract/2
  Integrator/1 -> "fhan "/2(v2), Integrator1/1  "v2"
  Subtract/1 -> "fhan "/1(v1)
  "fhan "/1(fhan) -> Integrator/1
  v0/1 -> Integrator1/2

== system New_FMS/Commander/Return/Velocity Commander/Lateral Acceleration/Included Angle ==
  vec1 : Inport
  vec2 : Inport  Port=2
  2D Cross Product : FMT_Model_Lib/Math/2D Cross Product
      settings: SourceProductName=FMT Toolbox
  Acos : Trigonometry  Operator=acos
  Constant4 : Constant  OutDataTypeStr=single
  Demux : Demux  Outputs=2
  Demux1 : Demux  Outputs=2
  Dot Product : DotProduct  InputSameDT=on  OutDataTypeStr=Inherit: Inherit via internal rule
  Multiply : Product
  Mux : Mux  Inputs=2
  Mux1 : Mux  Inputs=2
  Sign1 : Signum
  Switch2 : Switch  Criteria=u2 ~= 0
  Vector Normalize : FMT_Model_Lib/Math/Vector Normalize
      settings: SourceProductName=FMT Toolbox
  Vector Normalize1 : FMT_Model_Lib/Math/Vector Normalize
      settings: SourceProductName=FMT Toolbox
  angle_rad : Outport
  wires:
  Dot Product/1 -> Acos/1
  Demux1/1 -> Mux1/2
  Mux1/1 -> Vector Normalize/1
  Demux1/2 -> Mux1/1
  Sign1/1 -> Switch2/1, Switch2/2
  Vector Normalize1/1 -> Dot Product/2, 2D Cross Product/1
  Demux/2 -> Mux/1
  Vector Normalize/1 -> Dot Product/1, 2D Cross Product/2
  2D Cross Product/1 -> Sign1/1
  Multiply/1 -> angle_rad/1
  vec1/1 -> Demux1/1
  Demux/1 -> Mux/2
  Constant4/1 -> Switch2/3
  vec2/1 -> Demux/1
  Mux/1 -> Vector Normalize1/1
  Acos/1 -> Multiply/1
  Switch2/1 -> Multiply/2

== system New_FMS/Commander/Takeoff/Position Command/Controller/Brake Control ==
  Action Port : ActionPort  InitializeStates=reset  ActionType=case
  Brake Speed : Constant  Value=[0;0]  VectorParams1D=off  OutDataTypeStr=single
  uv_cmd_mPs : Outport
  wires:
  Brake Speed/1 -> uv_cmd_mPs/1

== system New_FMS/Commander/Takeoff/Position Command/Controller/Hold Control ==
  FMS_In : Inport
  Action Port : ActionPort  InitializeStates=reset  ActionType=case
  Bus Selector : BusSelector  OutputSignals=INS_Out.psi
  Bus_Selection : Subsystem
  Constant : Constant  Value=0  OutDataTypeStr=Inherit: Inherit via back propagation
  Delay : Delay  DelayLength=1  InitialConditionSource=Input port
      settings: InputPortMap=u0,p4
  Gain2 : Gain  Gain=FMS_PARAM.XY_P  OutDataTypeStr=single
  Multiply : Product  Multiplication=Matrix(*)
  Mux : Mux  Inputs=2
  Psi To DCM : FMT_Model_Lib/Transformation/Psi To DCM
      settings: SourceProductName=FMT Toolbox
  Selector : Selector  InputPortWidth=3  IndexOptions=Index vector (dialog)  Indices=[1 2]  OutputSizes=1
  Sum : Sum  Inputs=-+|
  uv_cmd_mPs : Outport
  wires:
  Gain2/1 -> uv_cmd_mPs/1
  Bus_Selection/1(xy_R_O_m) -> Sum/1, Delay/2  "xy_est_R"
  Sum/1 -> Mux/1  "xy_err_R"
  Delay/1 -> Delay/1, Sum/2  "xy_cmd_R"
  FMS_In/1 -> Bus Selector/1, Bus_Selection/1(FMS_In)
  Constant/1 -> Mux/2
  Psi To DCM/1 -> Multiply/1  "M_CO"
  Multiply/1 -> Selector/1
  Mux/1 -> Multiply/2
  Selector/1 -> Gain2/1
  Bus Selector/1 -> Psi To DCM/1  "<psi>"

== system New_FMS/Commander/Takeoff/Position Command/Controller/Move Control ==
  FMS_In : Inport
  Action Port : ActionPort  InitializeStates=reset  ActionType=case
  Bus Selector : BusSelector  OutputSignals=Pilot_Cmd_Proc.stick_pitch,Pilot_Cmd_Proc.stick_roll
  DeadZone : Subsystem  mask{th=FMS_PARAM.PITCH_DZ}
      mask prompts: th "Threshold"
      mask Display: disp('Dead Zone')
  DeadZone1 : Subsystem  mask{th=FMS_PARAM.ROLL_DZ}
      mask prompts: th "Threshold"
      mask Display: disp('Dead Zone')
  Gain6 : Gain  Gain=FMS_PARAM.VEL_XY_LIM  OutDataTypeStr=single
  Mux1 : Mux  Inputs=2
  TD : Subsystem
  uv_cmd_mPs : Outport
  wires:
  Gain6/1 -> TD/1(v)
  DeadZone/1(y) -> Mux1/1
  Bus Selector/1 -> DeadZone/1(u)  "<stick_pitch>"
  FMS_In/1 -> Bus Selector/1
  TD/1(v1) -> uv_cmd_mPs/1
  Bus Selector/2 -> DeadZone1/1(u)  "<stick_roll>"
  DeadZone1/1(y) -> Mux1/2
  Mux1/1 -> Gain6/1
